simulink model "pl6b"  (R2017b)
settings: Solver=VariableStepAuto  StartTime=0.0  StopTime=2.5  RelTol=1e-3
values from neighbouring files (symbols this model uses):
  A = [0 a12   0   0 ... (first row only)    [PreLab6a.m]
  Ak = A-B*K    [PreLab6a.m]
  Bk = B*K    [PreLab6a.m]
  ref = [0;0;0;0]    [PreLab6a.m]
undefined symbols (not defined in the file or in its folder): Cl, ic
settings Model: Creator=Jenny  LastModifiedBy=Jenny

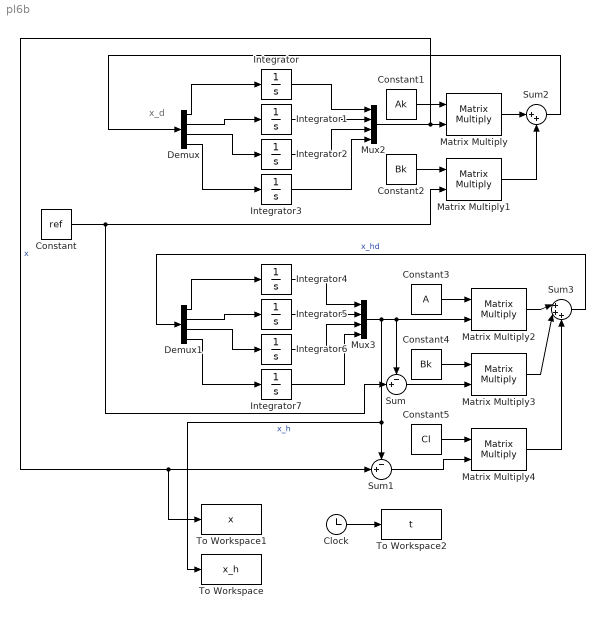
== system pl6b ==
  note: x_d
  Clock : Clock
  Constant : Constant  Value=ref
  Constant1 : Constant  Value=Ak
  Constant2 : Constant  Value=Bk
  Constant3 : Constant  Value=A
  Constant4 : Constant  Value=Bk
  Constant5 : Constant  Value=Cl
  Demux : Demux
  Demux1 : Demux
  Integrator : Integrator  InitialCondition=ic(1)
  Integrator1 : Integrator  InitialCondition=ic(2)
  Integrator2 : Integrator  InitialCondition=ic(3)
  Integrator3 : Integrator  InitialCondition=ic(4)
  Integrator4 : Integrator  InitialCondition=ic(1)
  Integrator5 : Integrator  InitialCondition=ic(2)
  Integrator6 : Integrator  InitialCondition=ic(3)
  Integrator7 : Integrator  InitialCondition=ic(4)
  Matrix Multiply{,1..4} (5 alike) : Product  Multiplication=Matrix(*)
  Mux2 : Mux
  Mux3 : Mux
  Sum : Sum  Inputs=-+|
  Sum1 : Sum  Inputs=-+|
  Sum2 : Sum  Inputs=|++
  Sum3 : Sum  Inputs=|+++
  To Workspace : ToWorkspace  VariableName=x_h  SampleTime=-1
  To Workspace1 : ToWorkspace  VariableName=x  SampleTime=-1
  To Workspace2 : ToWorkspace  VariableName=t  SampleTime=-1
  wires:
  Demux/1 -> Integrator/1
  Demux/4 -> Integrator3/1
  Demux/3 -> Integrator2/1
  Demux/2 -> Integrator1/1
  Sum3/1 -> Demux1/1  "x_hd"
  Demux1/3 -> Integrator6/1
  Demux1/4 -> Integrator7/1
  Demux1/2 -> Integrator5/1
  Demux1/1 -> Integrator4/1
  Integrator/1 -> Mux2/1
  Integrator1/1 -> Mux2/2
  Integrator2/1 -> Mux2/3
  Integrator3/1 -> Mux2/4
  Integrator4/1 -> Mux3/1
  Integrator5/1 -> Mux3/2
  Integrator6/1 -> Mux3/3
  Integrator7/1 -> Mux3/4
  Mux2/1 -> To Workspace1/1, Sum1/2, Matrix Multiply/2  "x"
  Constant1/1 -> Matrix Multiply/1
  Matrix Multiply/1 -> Sum2/1
  Constant2/1 -> Matrix Multiply1/1
  Constant/1 -> Sum/2, Matrix Multiply1/2
  Matrix Multiply1/1 -> Sum2/2
  Sum2/1 -> Demux/1
  Constant3/1 -> Matrix Multiply2/1
  Constant4/1 -> Matrix Multiply3/1
  Mux3/1 -> To Workspace/1, Sum1/1, Sum/1, Matrix Multiply2/2  "x_h"
  Matrix Multiply2/1 -> Sum3/1
  Matrix Multiply3/1 -> Sum3/2
  Sum/1 -> Matrix Multiply3/2
  Matrix Multiply4/1 -> Sum3/3
  Constant5/1 -> Matrix Multiply4/1
  Sum1/1 -> Matrix Multiply4/2
  Clock/1 -> To Workspace2/1
